simulink model "JOINTS_SPACE"  (R2021a)
settings: Solver=FixedStepAuto  StartTime=0.0  StopTime=30  FixedStep=0.01  RelTol=1e-3
model workspace: external: MATLAB File D:\OneDrive\STUDY\RIC LAB\PROJECT 6DOF\CODE\CODE 6DOF\10_SIMSCAPE\03\ROBOT_DataFile.m (data not in the file)
values from neighbouring files (symbols this model uses):
  circle = zeros(10/step+1,7)    [CIRCLE_01.m]
undefined symbols (not defined in the file or in its folder): smiData, X, Y, Z
libraries: sm_lib x36, nesl_utility x8
(part 1 of 2)
settings Model: Creator=TMP  LastModifiedBy=TMP
settings DataIOCC: SaveTime=off  ReturnWorkspaceOutputs=off

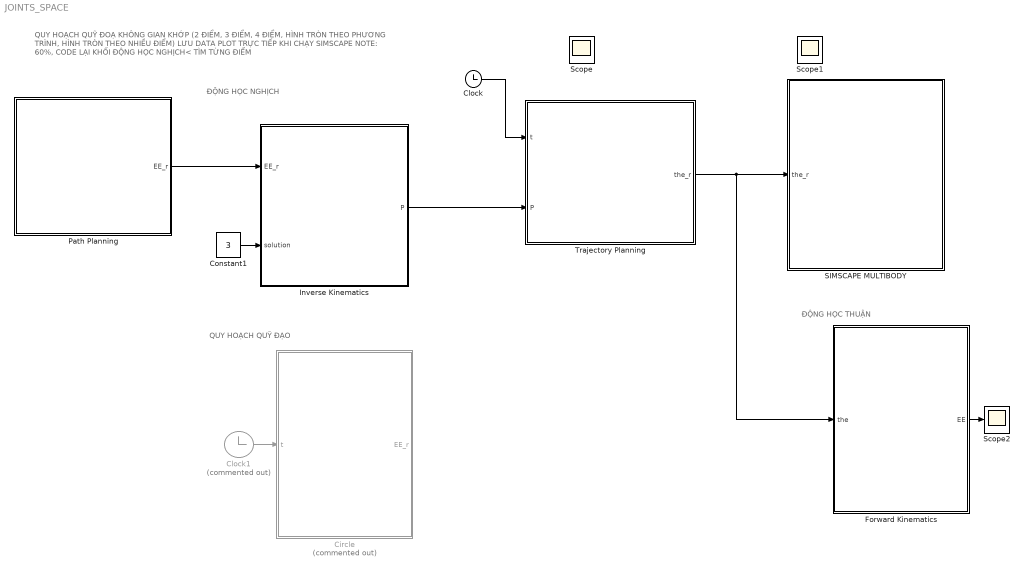
== system JOINTS_SPACE ==
  note: QUY HOẠCH QUỸ ĐOẠ KHÔNG GIAN KHỚP (2 ĐIỂM, 3 ĐIỂM, 4 ĐIỂM, HÌNH TRÒN THEO PHƯƠNG TRÌNH, HÌNH TRÒN THEO NHIỀU ĐIỂM)
      | LƯU DATA PLOT TRỰC TIẾP KHI CHẠY SIMSCAPE
      | NOTE: 60%, CODE LẠI KHỐI ĐỘNG HỌC NGHỊCH< TÌM TỪNG ĐIỂM
  note: ĐỘNG HỌC NGHỊCH
  note: QUY HOẠCH QUỸ ĐẠO
  note: ĐỘNG HỌC THUẬN
  Circle : MATLAB Function  Commented=on  TreatAsAtomicUnit=on
  Clock : Clock
  Clock1 : Clock  Commented=on
  Constant1 : Constant  Value=3
  Forward Kinematics : MATLAB Function  TreatAsAtomicUnit=on
  Inverse Kinematics : MATLAB Function  TreatAsAtomicUnit=on
  Path Planning : Subsystem
  SIMSCAPE MULTIBODY : Subsystem
  Scope : Scope
  Scope1 : Scope
  Scope2 : Scope
  Trajectory Planning : MATLAB Function  TreatAsAtomicUnit=on
  wires:
  Clock/1 -> Trajectory Planning/1(t)
  Constant1/1 -> Inverse Kinematics/2(solution)
  Clock1/1 -> Circle/1(t)
  Forward Kinematics/1(EE) -> Scope2/1
  Trajectory Planning/1(the_r) -> Forward Kinematics/1(the), SIMSCAPE MULTIBODY/1(the_r)
  Path Planning/1(EE_r) -> Inverse Kinematics/1(EE_r)
  Inverse Kinematics/1(P) -> Trajectory Planning/2(P)

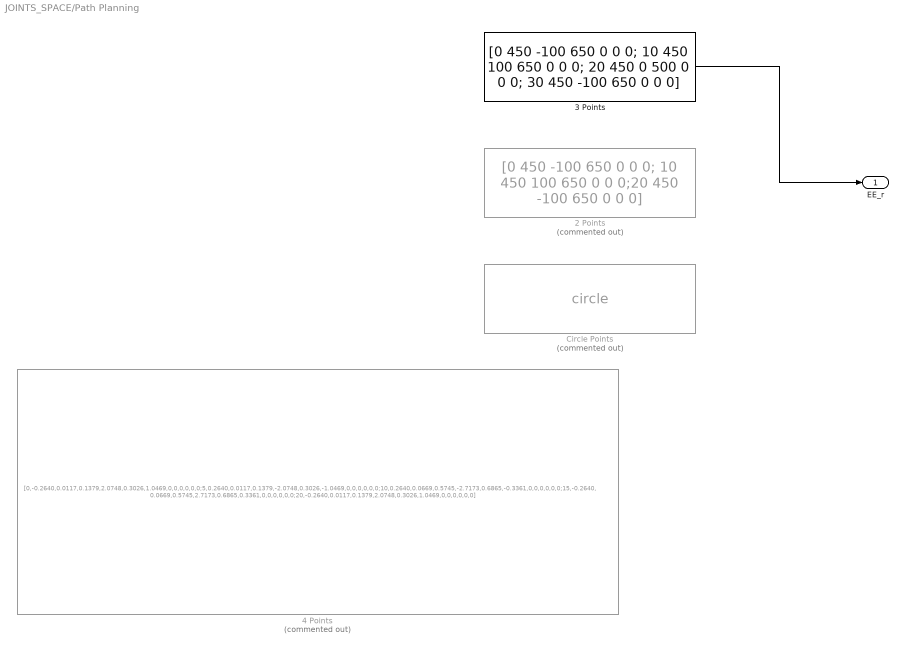
== system JOINTS_SPACE/Path Planning ==
  2 Points : Constant  Commented=on  Value=[0 450 -100 650 0 0 0; 10 450 100 650 0 0 0;20 450 -100 650 0 0 0]
  3 Points : Constant  Value=[0 450 -100 650 0 0 0; 10 450 100 650 0 0 0; 20 450 0 500 0 0 0; 30 450 -100 650 0 0 0]
  4 Points : Constant  Commented=on  Value=[0,-0.2640,0.0117,0.1379,2.0748,0.3026,1.0469,0,0,0,0,0,0;5,0.2640,0.0117,0.1379,-2.0748,0.3026,-1.0469,0,0,0,0,0,0;10,0.2640,0.0669,0.5745,-2.7173,0.6865,-0.3361,0,0,0,0,0,0;15,-0.2640, 0.0669,0.5745,2.7173,0.6865,0.3361,0,0,0,0,0,0;20,-0.2640,0.0117,0.1379,2.0748,0.3026,1.0469,0,0,0,0,0,0]
  Circle Points : Constant  Commented=on  Value=circle
  EE_r : Outport
  wires:
  3 Points/1 -> EE_r/1

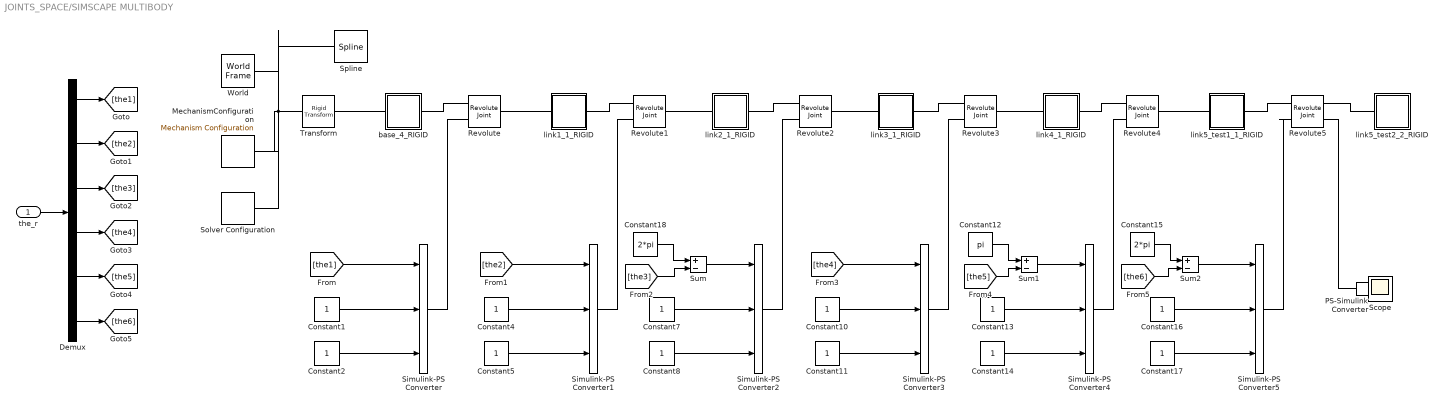
== system JOINTS_SPACE/SIMSCAPE MULTIBODY ==
  the_r : Inport
  Constant{1..2,4..5,7..8,10..11,13..14,16..17} (12 alike) : Constant
  Constant12 : Constant  Value=pi
  Constant15 : Constant  Value=2*pi
  Constant18 : Constant  Value=2*pi
  Demux : Demux  Outputs=6
  MechanismConfiguration : sm_lib/Utilities/Mechanism Configuration  UniformGravity=Constant  GravityVector=[0 -9.80665 0]  GravityVectorUnits=m/s^2  GravityUnits=m/s^2  LinearizationDelta=0.001  JointModeTransitionNonlinearIterations=2
  PS-Simulink Converter : nesl_utility/PS-Simulink Converter  PhysicalDomain=network_engine_domain  SubClassName=ps_output  LeftPortType=input  RightPortType=output  PseudoPeriodic=off  Frequencies=[]  Unit=inherit  AffineConversion=off
      settings: SourceProductBaseCode=PW,SS
  Revolute : sm_lib/Joints/Revolute Joint  JointMode=Normal  SenseConstraintForce=off  SenseConstraintForceX=off  SenseConstraintForceY=off  SenseConstraintForceZ=off  SenseConstraintTorque=off  SenseConstraintTorqueX=off  SenseConstraintTorqueY=off  SenseConstraintTorqueZ=off  SenseTotalForce=off  SenseTotalForceX=off  SenseTotalForceY=off  SenseTotalForceZ=off  SenseTotalTorque=off  SenseTotalTorqueX=off  SenseTotalTorqueY=off  SenseTotalTorqueZ=off  CompositeWrenchDir=FollowerOnBase  CompositeWrenchFrame=BaseFrame  EquilibriumPosition=0  EquilibriumPositionUnits=deg  SpringStiffness=0  SpringStiffnessUnits=N*m/deg  DampingCoefficient=0  DampingCoefficientUnits=N*m/(deg/s)  TorqueActuationMode=ComputedTorque  MotionActuationMode=InputMotion  SensePosition=off  SenseVelocity=off  SenseAcceleration=off  SenseTorqueForce=off  SenseLowerLimitTorqueForce=off  SenseUpperLimitTorqueForce=off  LowerLimitSpecify=off  LowerLimitBound=-90  LowerLimitBoundUnits=deg  LowerLimitStiffness=1e4  LowerLimitStiffnessUnits=N*m/deg  LowerLimitDamping=10  LowerLimitDampingUnits=N*m/(deg/s)  LowerLimitTransitionRegionWidth=0.1  LowerLimitTransitionRegionWidthUnits=deg  UpperLimitSpecify=off  UpperLimitBound=90  UpperLimitBoundUnits=deg  UpperLimitStiffness=1e4  UpperLimitStiffnessUnits=N*m/deg  UpperLimitDamping=10  UpperLimitDampingUnits=N*m/(deg/s)  UpperLimitTransitionRegionWidth=0.1  UpperLimitTransitionRegionWidthUnits=deg  PositionTargetSpecify=on  PositionTargetPriority=Low  PositionTargetValue=smiData.RevoluteJoint(2).Rz.Pos  PositionTargetValueUnits=deg  VelocityTargetSpecify=off  VelocityTargetPriority=High  VelocityTargetValue=0  VelocityTargetValueUnits=deg/s
  Revolute1 : sm_lib/Joints/Revolute Joint  JointMode=Normal  SenseConstraintForce=off  SenseConstraintForceX=off  SenseConstraintForceY=off  SenseConstraintForceZ=off  SenseConstraintTorque=off  SenseConstraintTorqueX=off  SenseConstraintTorqueY=off  SenseConstraintTorqueZ=off  SenseTotalForce=off  SenseTotalForceX=off  SenseTotalForceY=off  SenseTotalForceZ=off  SenseTotalTorque=off  SenseTotalTorqueX=off  SenseTotalTorqueY=off  SenseTotalTorqueZ=off  CompositeWrenchDir=FollowerOnBase  CompositeWrenchFrame=BaseFrame  EquilibriumPosition=0  EquilibriumPositionUnits=deg  SpringStiffness=0  SpringStiffnessUnits=N*m/deg  DampingCoefficient=0  DampingCoefficientUnits=N*m/(deg/s)  TorqueActuationMode=ComputedTorque  MotionActuationMode=InputMotion  SensePosition=off  SenseVelocity=off  SenseAcceleration=off  SenseTorqueForce=off  SenseLowerLimitTorqueForce=off  SenseUpperLimitTorqueForce=off  LowerLimitSpecify=off  LowerLimitBound=-90  LowerLimitBoundUnits=deg  LowerLimitStiffness=1e4  LowerLimitStiffnessUnits=N*m/deg  LowerLimitDamping=10  LowerLimitDampingUnits=N*m/(deg/s)  LowerLimitTransitionRegionWidth=0.1  LowerLimitTransitionRegionWidthUnits=deg  UpperLimitSpecify=off  UpperLimitBound=90  UpperLimitBoundUnits=deg  UpperLimitStiffness=1e4  UpperLimitStiffnessUnits=N*m/deg  UpperLimitDamping=10  UpperLimitDampingUnits=N*m/(deg/s)  UpperLimitTransitionRegionWidth=0.1  UpperLimitTransitionRegionWidthUnits=deg  PositionTargetSpecify=on  PositionTargetPriority=Low  PositionTargetValue=smiData.RevoluteJoint(1).Rz.Pos  PositionTargetValueUnits=deg  VelocityTargetSpecify=off  VelocityTargetPriority=High  VelocityTargetValue=0  VelocityTargetValueUnits=deg/s
  Revolute2 : sm_lib/Joints/Revolute Joint  JointMode=Normal  SenseConstraintForce=off  SenseConstraintForceX=off  SenseConstraintForceY=off  SenseConstraintForceZ=off  SenseConstraintTorque=off  SenseConstraintTorqueX=off  SenseConstraintTorqueY=off  SenseConstraintTorqueZ=off  SenseTotalForce=off  SenseTotalForceX=off  SenseTotalForceY=off  SenseTotalForceZ=off  SenseTotalTorque=off  SenseTotalTorqueX=off  SenseTotalTorqueY=off  SenseTotalTorqueZ=off  CompositeWrenchDir=FollowerOnBase  CompositeWrenchFrame=BaseFrame  EquilibriumPosition=0  EquilibriumPositionUnits=deg  SpringStiffness=0  SpringStiffnessUnits=N*m/deg  DampingCoefficient=0  DampingCoefficientUnits=N*m/(deg/s)  TorqueActuationMode=ComputedTorque  MotionActuationMode=InputMotion  SensePosition=off  SenseVelocity=off  SenseAcceleration=off  SenseTorqueForce=off  SenseLowerLimitTorqueForce=off  SenseUpperLimitTorqueForce=off  LowerLimitSpecify=off  LowerLimitBound=-90  LowerLimitBoundUnits=deg  LowerLimitStiffness=1e4  LowerLimitStiffnessUnits=N*m/deg  LowerLimitDamping=10  LowerLimitDampingUnits=N*m/(deg/s)  LowerLimitTransitionRegionWidth=0.1  LowerLimitTransitionRegionWidthUnits=deg  UpperLimitSpecify=off  UpperLimitBound=90  UpperLimitBoundUnits=deg  UpperLimitStiffness=1e4  UpperLimitStiffnessUnits=N*m/deg  UpperLimitDamping=10  UpperLimitDampingUnits=N*m/(deg/s)  UpperLimitTransitionRegionWidth=0.1  UpperLimitTransitionRegionWidthUnits=deg  PositionTargetSpecify=on  PositionTargetPriority=Low  PositionTargetValue=smiData.RevoluteJoint(3).Rz.Pos  PositionTargetValueUnits=deg  VelocityTargetSpecify=off  VelocityTargetPriority=High  VelocityTargetValue=0  VelocityTargetValueUnits=deg/s
  Revolute3 : sm_lib/Joints/Revolute Joint  JointMode=Normal  SenseConstraintForce=off  SenseConstraintForceX=off  SenseConstraintForceY=off  SenseConstraintForceZ=off  SenseConstraintTorque=off  SenseConstraintTorqueX=off  SenseConstraintTorqueY=off  SenseConstraintTorqueZ=off  SenseTotalForce=off  SenseTotalForceX=off  SenseTotalForceY=off  SenseTotalForceZ=off  SenseTotalTorque=off  SenseTotalTorqueX=off  SenseTotalTorqueY=off  SenseTotalTorqueZ=off  CompositeWrenchDir=FollowerOnBase  CompositeWrenchFrame=BaseFrame  EquilibriumPosition=0  EquilibriumPositionUnits=deg  SpringStiffness=0  SpringStiffnessUnits=N*m/deg  DampingCoefficient=0  DampingCoefficientUnits=N*m/(deg/s)  TorqueActuationMode=ComputedTorque  MotionActuationMode=InputMotion  SensePosition=off  SenseVelocity=off  SenseAcceleration=off  SenseTorqueForce=off  SenseLowerLimitTorqueForce=off  SenseUpperLimitTorqueForce=off  LowerLimitSpecify=off  LowerLimitBound=-90  LowerLimitBoundUnits=deg  LowerLimitStiffness=1e4  LowerLimitStiffnessUnits=N*m/deg  LowerLimitDamping=10  LowerLimitDampingUnits=N*m/(deg/s)  LowerLimitTransitionRegionWidth=0.1  LowerLimitTransitionRegionWidthUnits=deg  UpperLimitSpecify=off  UpperLimitBound=90  UpperLimitBoundUnits=deg  UpperLimitStiffness=1e4  UpperLimitStiffnessUnits=N*m/deg  UpperLimitDamping=10  UpperLimitDampingUnits=N*m/(deg/s)  UpperLimitTransitionRegionWidth=0.1  UpperLimitTransitionRegionWidthUnits=deg  PositionTargetSpecify=on  PositionTargetPriority=Low  PositionTargetValue=smiData.RevoluteJoint(4).Rz.Pos  PositionTargetValueUnits=deg  VelocityTargetSpecify=off  VelocityTargetPriority=High  VelocityTargetValue=0  VelocityTargetValueUnits=deg/s
  Revolute4 : sm_lib/Joints/Revolute Joint  JointMode=Normal  SenseConstraintForce=off  SenseConstraintForceX=off  SenseConstraintForceY=off  SenseConstraintForceZ=off  SenseConstraintTorque=off  SenseConstraintTorqueX=off  SenseConstraintTorqueY=off  SenseConstraintTorqueZ=off  SenseTotalForce=off  SenseTotalForceX=off  SenseTotalForceY=off  SenseTotalForceZ=off  SenseTotalTorque=off  SenseTotalTorqueX=off  SenseTotalTorqueY=off  SenseTotalTorqueZ=off  CompositeWrenchDir=FollowerOnBase  CompositeWrenchFrame=BaseFrame  EquilibriumPosition=0  EquilibriumPositionUnits=deg  SpringStiffness=0  SpringStiffnessUnits=N*m/deg  DampingCoefficient=0  DampingCoefficientUnits=N*m/(deg/s)  TorqueActuationMode=ComputedTorque  MotionActuationMode=InputMotion  SensePosition=off  SenseVelocity=off  SenseAcceleration=off  SenseTorqueForce=off  SenseLowerLimitTorqueForce=off  SenseUpperLimitTorqueForce=off  LowerLimitSpecify=off  LowerLimitBound=-90  LowerLimitBoundUnits=deg  LowerLimitStiffness=1e4  LowerLimitStiffnessUnits=N*m/deg  LowerLimitDamping=10  LowerLimitDampingUnits=N*m/(deg/s)  LowerLimitTransitionRegionWidth=0.1  LowerLimitTransitionRegionWidthUnits=deg  UpperLimitSpecify=off  UpperLimitBound=90  UpperLimitBoundUnits=deg  UpperLimitStiffness=1e4  UpperLimitStiffnessUnits=N*m/deg  UpperLimitDamping=10  UpperLimitDampingUnits=N*m/(deg/s)  UpperLimitTransitionRegionWidth=0.1  UpperLimitTransitionRegionWidthUnits=deg  PositionTargetSpecify=on  PositionTargetPriority=Low  PositionTargetValue=smiData.RevoluteJoint(5).Rz.Pos  PositionTargetValueUnits=deg  VelocityTargetSpecify=off  VelocityTargetPriority=High  VelocityTargetValue=0  VelocityTargetValueUnits=deg/s
  Revolute5 : sm_lib/Joints/Revolute Joint  JointMode=Normal  SenseConstraintForce=off  SenseConstraintForceX=off  SenseConstraintForceY=off  SenseConstraintForceZ=off  SenseConstraintTorque=off  SenseConstraintTorqueX=off  SenseConstraintTorqueY=off  SenseConstraintTorqueZ=off  SenseTotalForce=off  SenseTotalForceX=off  SenseTotalForceY=off  SenseTotalForceZ=off  SenseTotalTorque=off  SenseTotalTorqueX=off  SenseTotalTorqueY=off  SenseTotalTorqueZ=off  CompositeWrenchDir=FollowerOnBase  CompositeWrenchFrame=BaseFrame  EquilibriumPosition=0  EquilibriumPositionUnits=deg  SpringStiffness=0  SpringStiffnessUnits=N*m/deg  DampingCoefficient=0  DampingCoefficientUnits=N*m/(deg/s)  TorqueActuationMode=ComputedTorque  MotionActuationMode=InputMotion  SensePosition=on  SenseVelocity=off  SenseAcceleration=off  SenseTorqueForce=off  SenseLowerLimitTorqueForce=off  SenseUpperLimitTorqueForce=off  LowerLimitSpecify=off  LowerLimitBound=-90  LowerLimitBoundUnits=deg  LowerLimitStiffness=1e4  LowerLimitStiffnessUnits=N*m/deg  LowerLimitDamping=10  LowerLimitDampingUnits=N*m/(deg/s)  LowerLimitTransitionRegionWidth=0.1  LowerLimitTransitionRegionWidthUnits=deg  UpperLimitSpecify=off  UpperLimitBound=90  UpperLimitBoundUnits=deg  UpperLimitStiffness=1e4  UpperLimitStiffnessUnits=N*m/deg  UpperLimitDamping=10  UpperLimitDampingUnits=N*m/(deg/s)  UpperLimitTransitionRegionWidth=0.1  UpperLimitTransitionRegionWidthUnits=deg  PositionTargetSpecify=on  PositionTargetPriority=Low  PositionTargetValue=smiData.RevoluteJoint(6).Rz.Pos  PositionTargetValueUnits=deg  VelocityTargetSpecify=off  VelocityTargetPriority=High  VelocityTargetValue=0  VelocityTargetValueUnits=deg/s
  Scope : Scope
  Simulink-PS Converter{,1..5} (6 alike) : nesl_utility/Simulink-PS Converter  PhysicalDomain=network_engine_domain  SubClassName=ps_input  LeftPortType=input  RightPortType=output  PseudoPeriodic=off  Frequencies=[]  NoiseDistribution=none  NoiseParameters=[]  Unit=1  AffineConversion=off  FilteringAndDerivatives=provide  SimscapeFilterOrder=1  InputFilterTimeConstant=0.001  UdotUserProvided=2
      settings: SourceProductBaseCode=PW,SS
  Solver Configuration : nesl_utility/Solver Configuration  PhysicalDomain=network_engine_domain  SubClassName=solver  LeftPortType=input  RightPortType=generic  Tones=[]  Harmonics=[]  SimulateNoise=off  Profile=off  UseLocalSampling=off  EnableSwitchedLinearOptims=on  FrequencyDomain=off  UseCCode=off  RelTol=0.001  AbsTol=1e-06  MinStep=1e-09  ToWorkspace=off  RevertToSquareIcSolve=off  NumHomotopyIterations=100  PhasorMode=off  PhasorModeNumHarmonics=1  DoDC=off  ResidualTolerance=1e-09  UseLocalSolver=off  LocalSolverChoice=NE_BACKWARD_EULER_ADVANCER  LocalSolverSampleTime=0.001  DoFixedCost=off  MaxNonlinIter=3  MaxModeIter=2  ComputeImpulses=off  ImpulseIterations=2  LinearAlgebra=auto  EquationFormulation=NE_TIME_EF  DelaysMemoryBudget=1024  AutomaticFiltering=on  FilteringTimeConstant=0.001  PartitionStorageMethod=AS_NEEDED  PartitionMemoryBudget=1024  PartitionMethod=ROBUST
      settings: SourceProductBaseCode=PW,SS
  Spline : sm_lib/Curves and Surfaces/Spline  GraphicAmbientColor=[0.15 0.15 0.15 1.0]  GraphicDiffuseColor=[0.0 0.0 0.0]  DataPoints=|  DataPointsUnits=mm  GraphicEmissiveColor=[0.0 0.0 0.0 1.0]  EndConditionType=Natural  MarkerShape=Sphere  MarkerSize=10  GraphicType=FromGeometry  GraphicOpacity=1.0  GraphicShininess=75  GraphicSpecularColor=[0.5 0.5 0.5 1.0]  GraphicVisPropType=SimpleVisualProperties
      | [450.0000 -100.0000  650.0000
      |   450.0025  -99.9863  649.9959
      |   450.0101  -99.9452  649.9836
      |   450.0226  -99.8770  649.9633
      |   450.0400  -99.7820  649.9349
      |   450.0623  -99.6603  649.8985
      |   450.0893  -99.5124  649.8541
      |   450.1211  -99.3383  649.8018
      |   450.1574  -99.1384  649.7416
      |   450.1982  -98.9130  649.6736
      |   450.2434  -98.6623  649.5977
      |   450.2929  -98.3867  649.5141
      |   450.3465  -98.0864  649.4226
      |   450.4043  -97.7618  649.3234
      |   450.4659  -97.4131  649.2165
      |   450.5313  -97.0408  649.1017
      |   450.6004  -96.6450  648.9793
      |   450.6730  -96.2262  648.8491
      |   450.7490  -95.7847  648.7113
      |   450.8283  -95.3209  648.5657
      |   450.9106  -94.8350  648.4124
      |   450.9958  -94.3276  648.2514
      |   451.0837  -93.7988  648.0827
      |   451.1743  -93.2491  647.9063
      |   451.2673  -92.6789  647.7223
      |   451.3626  -92.0886  647.5305
      |   451.4600  -91.4785  647.3311
      |   451.5593  -90.8490  647.1240
      |   451.6604  -90.2006  646.9093
      |   451.7631  -89.5337  646.6869
      |   451.8672  -88.8486  646.4570
      |   451.9725  -88.1458  646.2194
      |   452.0789  -87.4257  645.9743
      |   452.1862  -86.6887  645.7216
      |   452.2942  -85.9353  645.4614
      |   452.4027  -85.1659  645.1937
      |   452.5117  -84.3810  644.9186
      |   452.6208  -83.5809  644.6361
      |   452.7300  -82.7662  644.3462
      |   452.8390  -81.9372  644.0491
      |   452.9478  -81.0945  643.7447
      |   453.0561  -80.2385  643.4332
      |   453.1637  -79.3697  643.1146
      |   453.2706  -78.4885  642.7891
      |   453.3766  -77.5954  642.4566
      |   453.4815  -76.6908  642.1173
      |   453.5851  -75.7753  641.7713
      |   453.6874  -74.8494  641.4188
      |   453.7882  -73.9134  641.0598
      |   453.8874  -72.9678  640.6944
      |   453.9847  -72.0133  640.3228
      |   454.0802  -71.0501  639.9452
      |   454.1737  -70.0788  639.5617
      |   454.2650  -69.0999  639.1725
      |   454.3542  -68.1138  638.7777
      |   454.4410  -67.1210  638.3775
      |   454.5253  -66.1219  637.9721
      |   454.6072  -65.1171  637.5618
      |   454.6864  -64.1070  637.1466
      |   454.7630  -63.0921  636.7270
      |   454.8368  -62.0728  636.3029
      |   454.9078  -61.0495  635.8748
      |   454.9759  -60.0228  635.4428
      |   455.0412  -58.9930  635.0073
      |   455.1034  -57.9605  634.5684
      |   455.1627  -56.9259  634.1264
      |   455.2190  -55.8895  633.6817
      |   455.2722  -54.8517  633.2345
      |   455.3223  -53.8130  632.7851
      |   455.3694  -52.7737  632.3338
      |   455.4134  -51.7343  631.8810
      |   455.4544  -50.6950  631.4269
      |   455.4923  -49.6563  630.9719
      |   455.5272  -48.6185  630.5163
      |   455.5591  -47.5820  630.0605
      |   455.5881  -46.5471  629.6048
      |   455.6141  -45.5141  629.1496
      |   455.6373  -44.4833  628.6952
      |   455.6576  -43.4551  628.2420
      |   455.6752  -42.4296  627.7904
      |   455.6901  -41.4073  627.3407
      |   455.7023  -40.3883  626.8933
      |   455.7121  -39.3728  626.4487
      |   455.7193  -38.3611  626.0072
      |   455.7242  -37.3535  625.5691
      |   455.7268  -36.3501  625.1349
      |   455.7273  -35.3510  624.7050
      |   455.7256  -34.3565  624.2798
      |   455.7220  -33.3667  623.8596
      |   455.7164  -32.3818  623.4448
      |   455.7092  -31.4018  623.0359
      |   455.7003  -30.4269  622.6333
      |   455.6898  -29.4571  622.2372
      |   455.6779  -28.4925  621.8481
      |   455.6648  -27.5332  621.4665
      |   455.6504  -26.5792  621.0926
      |   455.6350  -25.6305  620.7268
      |   455.6187  -24.6872  620.3696
      |   455.6016  -23.7491  620.0212
      |   455.5838  -22.8164  619.6820
      |   455.5655  -21.8888  619.3525
      |   455.5467  -20.9665  619.0328
      |   455.5276  -20.0493  618.7234
      |   455.5084  -19.1371  618.4246
      |   455.4890  -18.2298  618.1367
      |   455.4697  -17.3273  617.8600
      |   455.4505  -16.4295  617.5948
      |   455.4316  -15.5363  617.3414
      |   455.4131  -14.6473  617.1001
      |   455.3950  -13.7626  616.8711
      |   455.3775  -12.8819  616.6546
      |   455.3607  -12.0050  616.4510
      |   455.3446  -11.1318  616.2604
      |   455.3294  -10.2619  616.0831
      |   455.3150   -9.3952  615.9192
      |   455.3017   -8.5315  615.7689
      |   455.2894   -7.6705  615.6325
      |   455.2783   -6.8119  615.5100
      |   455.2683   -5.9555  615.4015
      |   455.2595   -5.1011  615.3073
      |   455.2521   -4.2483  615.2274
      |   455.2459   -3.3970  615.1619
      |   455.2411   -2.5467  615.1109
      |   455.2376   -1.6974  615.0744
      |   455.2355   -0.8485  615.0525
      |   455.2348   -0.0000  615.0452
      |   455.2355    0.8485  615.0525
      |   455.2376    1.6974  615.0744
      |   455.2411    2.5467  615.1109
      |   455.2459    3.3970  615.1619
      |   455.2521    4.2483  615.2274
      |   455.2595    5.1011  615.3073
      |   455.2683    5.9555  615.4015
      |   455.2783    6.8119  615.5100
      |   455.2894    7.6705  615.6325
      |   455.3017    8.5315  615.7689
      |   455.3150    9.3952  615.9192
      |   455.3294   10.2619  616.0831
      |   455.3446   11.1318  616.2604
      |   455.3607   12.0050  616.4510
      |   455.3775   12.8819  616.6546
      |   455.3950   13.7626  616.8711
      |   455.4131   14.6473  617.1001
      |   455.4316   15.5363  617.3414
      |   455.4505   16.4295  617.5948
      |   455.4697   17.3273  617.8600
      |   455.4890   18.2298  618.1367
      |   455.5084   19.1371  618.4246
      |   455.5276   20.0493  618.7234
      |   455.5467   20.9665  619.0328
      |   455.5655   21.8888  619.3525
      |   455.5838   22.8164  619.6820
      |   455.6016   23.7491  620.0212
      |   455.6187   24.6872  620.3696
      |   455.6350   25.6305  620.7268
      |   455.6504   26.5792  621.0926
      |   455.6648   27.5332  621.4665
      |   455.6779   28.4925  621.8481
      |   455.6898   29.4571  622.2372
      |   455.7003   30.4269  622.6333
      |   455.7092   31.4018  623.0359
      |   455.7164   32.3818  623.4448
      |   455.7220   33.3667  623.8596
      |   455.7256   34.3565  624.2798
      |   455.7273   35.3510  624.7050
      |   455.7268   36.3501  625.1349
      |   455.7242   37.3535  625.5691
      |   455.7193   38.3611  626.0072
      |   455.7121   39.3728  626.4487
      |   455.7023   40.3883  626.8933
      |   455.6901   41.4073  627.3407
      |   455.6752   42.4296  627.7904
      |   455.6576   43.4551  628.2420
      |   455.6373   44.4833  628.6952
      |   455.6141   45.5141  629.1496
      |   455.5881   46.5471  629.6048
      |   455.5591   47.5820  630.0605
      |   455.5272   48.6185  630.5163
      |   455.4923   49.6563  630.9719
      |   455.4544   50.6950  631.4269
      |   455.4134   51.7343  631.8810
      |   455.3694   52.7737  632.3338
      |   455.3223   53.8130  632.7851
      |   455.2722   54.8517  633.2345
      |   455.2190   55.8895  633.6817
      |   455.1627   56.9259  634.1264
      |   455.1034   57.9605  634.5684
      |   455.0412   58.9930  635.0073
      |   454.9759   60.0228  635.4428
      |   454.9078   61.0495  635.8748
      |   454.8368   62.0728  636.3029
      |   454.7630   63.0921  636.7270
      |   454.6864   64.1070  637.1466
      |   454.6072   65.1171  637.5618
      |   454.5253   66.1219  637.9721
      |   454.4410   67.1210  638.3775
      |   454.3542   68.1138  638.7777
      |   454.2650   69.0999  639.1725
      |   454.1737   70.0788  639.5617
      |   454.0802   71.0501  639.9452
      |   453.9847   72.0133  640.3228
      |   453.8874   72.9678  640.6944
      |   453.7882   73.9134  641.0598
      |   453.6874   74.8494  641.4188
      |   453.5851   75.7753  641.7713
      |   453.4815   76.6908  642.1173
      |   453.3766   77.5954  642.4566
      |   453.2706   78.4885  642.7891
      |   453.1637   79.3697  643.1146
      |   453.0561   80.2385  643.4332
      |   452.9478   81.0945  643.7447
      |   452.8390   81.9372  644.0491
      |   452.7300   82.7662  644.3462
      |   452.6208   83.5809  644.6361
      |   452.5117   84.3810  644.9186
      |   452.4027   85.1659  645.1937
      |   452.2942   85.9353  645.4614
      |   452.1862   86.6887  645.7216
      |   452.0789   87.4257  645.9743
      |   451.9725   88.1458  646.2194
      |   451.8672   88.8486  646.4570
      |   451.7631   89.5337  646.6869
      |   451.6604   90.2006  646.9093
      |   451.5593   90.8490  647.1240
      |   451.4600   91.4785  647.3311
      |   451.3626   92.0886  647.5305
      |   451.2673   92.6789  647.7223
      |   451.1743   93.2491  647.9063
      |   451.0837   93.7988  648.0827
      |   450.9958   94.3276  648.2514
      |   450.9106   94.8350  648.4124
      |   450.8283   95.3209  648.5657
      |   450.7490   95.7847  648.7113
      |   450.6730   96.2262  648.8491
      |   450.6004   96.6450  648.9793
      |   450.5313   97.0408  649.1017
      |   450.4659   97.4131  649.2165
      |   450.4043   97.7618  649.3234
      |   450.3465   98.0864  649.4226
      |   450.2929   98.3867  649.5141
      |   450.2434   98.6623  649.5977
      |   450.1982   98.9130  649.6736
      |   450.1574   99.1384  649.7416
      |   450.1211   99.3383  649.8018
      |   450.0893   99.5124  649.8541
      |   450.0623   99.6603  649.8985
      |   450.0400   99.7820  649.9349
      |   450.0226   99.8770  649.9633
      |   450.0101   99.9452  649.9836
      |   450.0025   99.9863  649.9959
      |   450.0000  100.0000  650.0000
      |   450.0024   99.9905  649.9865
      |   450.0095   99.9621  649.9460
      |   450.0212   99.9150  649.8788
      |   450.0376   99.8494  649.7850
      |   450.0584   99.7654  649.6648
      |   450.0837   99.6633  649.5183
      |   450.1133   99.5431  649.3458
      |   450.1471   99.4053  649.1473
      |   450.1850   99.2499  648.9230
      |   450.2268   99.0771  648.6729
      |   450.2725   98.8873  648.3972
      |   450.3217   98.6807  648.0959
      |   450.3745   98.4575  647.7691
      |   450.4306   98.2179  647.4170
      |   450.4898   97.9623  647.0395
      |   450.5519   97.6910  646.6367
      |   450.6167   97.4041  646.2087
      |   450.6841   97.1021  645.7555
      |   450.7538   96.7852  645.2771
      |   450.8255   96.4538  644.7736
      |   450.8991   96.1081  644.2451
      |   450.9743   95.7486  643.6915
      |   451.0509   95.3755  643.1128
      |   451.1285   94.9893  642.5091
      |   451.2069   94.5903  641.8805
      |   451.2860   94.1789  641.2269
      |   451.3652   93.7555  640.5483
      |   451.4445   93.3205  639.8449
      |   451.5235   92.8743  639.1166
      |   451.6018   92.4174  638.3634
      |   451.6793   91.9503  637.5854
      |   451.7556   91.4733  636.7827
      |   451.8303   90.9869  635.9553
      |   451.9032   90.4917  635.1032
      |   451.9740   89.9881  634.2266
      |   452.0423   89.4767  633.3255
      |   452.1077   88.9579  632.4000
      |   452.1701   88.4323  631.4501
      |   452.2290   87.9005  630.4761
      |   452.2841   87.3631  629.4780
      |   452.3351   86.8205  628.4560
      |   452.3816   86.2734  627.4102
      |   452.4234   85.7224  626.3408
      |   452.4600   85.1680  625.2480
      |   452.4913   84.6110  624.1320
      |   452.5167   84.0520  622.9930
      |   452.5361   83.4915  621.8313
      |   452.5490   82.9303  620.6471
      |   452.5553   82.3689  619.4407
      |   452.5545   81.8082  618.2124
      |   452.5464   81.2486  616.9626
      |   452.5307   80.6910  615.6916
      |   452.5071   80.1361  614.3998
      |   452.4753   79.5844  613.0876
      |   452.4351   79.0368  611.7554
      |   452.3862   78.4939  610.4037
      |   452.3283   77.9564  609.0330
      |   452.2613   77.4250  607.6438
      |   452.1848   76.9005  606.2365
      |   452.0988   76.3835  604.8119
      |   452.0030   75.8748  603.3704
      |   451.8972   75.3750  601.9127
      |   451.7813   74.8849  600.4394
      |   451.6551   74.4051  598.9513
      |   451.5186   73.9363  597.4490
      |   451.3715   73.4792  595.9332
      |   451.2140   73.0345  594.4048
      |   451.0458   72.6027  592.8645
      |   450.8669   72.1846  591.3131
      |   450.6774   71.7808  589.7515
      |   450.4772   71.3918  588.1805
      |   450.2663   71.0183  586.6011
      |   450.0449   70.6607  585.0141
      |   449.8130   70.3197  583.4205
      |   449.5707   69.9958  581.8213
      |   449.3181   69.6895  580.2175
      |   449.0554   69.4011  578.6100
      |   448.7827   69.1313  576.9999
      |   448.5003   68.8803  575.3883
      |   448.2085   68.6486  573.7761
      |   447.9074   68.4365  572.1645
      |   447.5974   68.2443  570.5546
      |   447.2787   68.0722  568.9475
      |   446.9518   67.9206  567.3443
      |   446.6170   67.7897  565.7461
      |   446.2746   67.6794  564.1541
      |   445.9251   67.5901  562.5693
      |   445.5690   67.5218  560.9930
      |   445.2067   67.4744  559.4263
      |   444.8386   67.4480  557.8702
      |   444.4654   67.4426  556.3260
      |   444.0876   67.4579  554.7947
      |   443.7056   67.4939  553.2776
      |   443.3201   67.5504  551.7756
      |   442.9318   67.6271  550.2899
      |   442.5411   67.7237  548.8216
      |   442.1488   67.8399  547.3718
      |   441.7554   67.9752  545.9414
      |   441.3617   68.1293  544.5315
      |   440.9683   68.3016  543.1432
      |   440.5759   68.4916  541.7773
      |   440.1852   68.6988  540.4349
      |   439.7969   68.9224  539.1169
      |   439.4117   69.1618  537.8240
      |   439.0303   69.4163  536.5572
      |   438.6534   69.6851  535.3174
      |   438.2818   69.9674  534.1051
      |   437.9162   70.2623  532.9213
      |   437.5572   70.5689  531.7665
      |   437.2055   70.8864  530.6415
      |   436.8620   71.2136  529.5467
      |   436.5272   71.5497  528.4829
      |   436.2018   71.8935  527.4503
      |   435.8865   72.2440  526.4496
      |   435.5819   72.6001  525.4811
      |   435.2888   72.9607  524.5452
      |   435.0076   73.3245  523.6421
      |   434.7389   73.6904  522.7720
      |   434.4834   74.0571  521.9353
      |   434.2416   74.4236  521.1319
      |   434.0140   74.7885  520.3620
      |   433.8011   75.1505  519.6256
      |   433.6034   75.5085  518.9226
      |   433.4212   75.8611  518.2530
      |   433.2550   76.2070  517.6166
      |   433.1052   76.5451  517.0132
      |   432.9720   76.8741  516.4425
      |   432.8558   77.1925  515.9043
      |   432.7569   77.4994  515.3980
      |   432.6754   77.7932  514.9235
      |   432.6115   78.0730  514.4801
      |   432.5655   78.3373  514.0673
      |   432.5373   78.5851  513.6846
      |   432.5271   78.8151  513.3314
      |   432.5348   79.0263  513.0070
      |   432.5605   79.2175  512.7107
      |   432.6041   79.3876  512.4417
      |   432.6655   79.5355  512.1993
      |   432.7446   79.6603  511.9827
      |   432.8411   79.7610  511.7909
      |   432.9550   79.8367  511.6232
      |   433.0859   79.8864  511.4786
      |   433.2334   79.9093  511.3561
      |   433.3974   79.9047  511.2547
      |   433.5775   79.8717  511.1736
      |   433.7731   79.8098  511.1116
      |   433.9840   79.7181  511.0677
      |   434.2096   79.5963  511.0409
      |   434.4494   79.4437  511.0301
      |   434.7029   79.2598  511.0343
      |   434.9696   79.0443  511.0523
      |   435.2488   78.7968  511.0831
      |   435.5400   78.5169  511.1255
      |   435.8425   78.2046  511.1786
      |   436.1557   77.8595  511.2412
      |   436.4788   77.4817  511.3123
      |   436.8113   77.0709  511.3908
      |   437.1524   76.6273  511.4756
      |   437.5014   76.1509  511.5656
      |   437.8575   75.6418  511.6600
      |   438.2201   75.1003  511.7576
      |   438.5884   74.5265  511.8575
      |   438.9615   73.9208  511.9586
      |   439.3389   73.2836  512.0602
      |   439.7197   72.6152  512.1611
      |   440.1031   71.9162  512.2607
      |   440.4885   71.1870  512.3579
      |   440.8751   70.4283  512.4520
      |   441.2621   69.6406  512.5422
      |   441.6488   68.8247  512.6277
      |   442.0345   67.9813  512.7079
      |   442.4186   67.1111  512.7819
      |   442.8002   66.2149  512.8492
      |   443.1788   65.2937  512.9092
      |   443.5537   64.3483  512.9612
      |   443.9243   63.3796  513.0048
      |   444.2899   62.3885  513.0395
      |   444.6499   61.3762  513.0648
      |   445.0039   60.3435  513.0803
      |   445.3512   59.2916  513.0856
      |   445.6914   58.2215  513.0805
      |   446.0239   57.1343  513.0646
      |   446.3483   56.0311  513.0377
      |   446.6642   54.9131  512.9995
      |   446.9711   53.7814  512.9501
      |   447.2688   52.6372  512.8891
      |   447.5567   51.4816  512.8166
      |   447.8348   50.3158  512.7324
      |   448.1026   49.1411  512.6367
      |   448.3599   47.9585  512.5294
      |   448.6065   46.7693  512.4107
      |   448.8423   45.5748  512.2805
      |   449.0671   44.3759  512.1392
      |   449.2807   43.1741  511.9868
      |   449.4830   41.9703  511.8235
      |   449.6742   40.7659  511.6497
      |   449.8540   39.5620  511.4656
      |   450.0225   38.3597  511.2715
      |   450.1797   37.1601  511.0677
      |   450.3257   35.9644  510.8547
      |   450.4607   34.7738  510.6327
      |   450.5846   33.5892  510.4022
      |   450.6977   32.4118  510.1636
      |   450.8001   31.2426  509.9175
      |   450.8921   30.0827  509.6642
      |   450.9738   28.9330  509.4043
      |   451.0456   27.7946  509.1383
      |   451.1075   26.6685  508.8667
      |   451.1601   25.5556  508.5900
      |   451.2035   24.4568  508.3088
      |   451.2380   23.3731  508.0237
      |   451.2641   22.3052  507.7353
      |   451.2821   21.2542  507.4441
      |   451.2923   20.2207  507.1508
      |   451.2952   19.2057  506.8558
      |   451.2911   18.2098  506.5600
      |   451.2805   17.2339  506.2638
      |   451.2637   16.2787  505.9678
      |   451.2412   15.3449  505.6727
      |   451.2134   14.4333  505.3791
      |   451.1808   13.5443  505.0877
      |   451.1438   12.6788  504.7989
      |   451.1029   11.8374  504.5134
      |   451.0584   11.0206  504.2319
      |   451.0109   10.2290  503.9548
      |   450.9608    9.4631  503.6829
      |   450.9085    8.7237  503.4166
      |   450.8545    8.0110  503.1566
      |   450.7993    7.3257  502.9034
      |   450.7431    6.6683  502.6575
      |   450.6865    6.0392  502.4196
      |   450.6299    5.4389  502.1900
      |   450.5737    4.8677  501.9694
      |   450.5183    4.3262  501.7583
      |   450.4640    3.8148  501.5570
      |   450.4113    3.3338  501.3661
      |   450.3604    2.8837  501.1861
      |   450.3118    2.4648  501.0173
      |   450.2657    2.0775  500.8602
      |   450.2225    1.7222  500.7152
      |   450.1824    1.3992  500.5826
      |   450.1457    1.1088  500.4628
      |   450.1127    0.8514  500.3561
      |   450.0835    0.6273  500.2629
      |   450.0585    0.4369  500.1833
      |   450.0377    0.2804  500.1178
      |   450.0213    0.1582  500.0665
      |   450.0095    0.0705  500.0297
      |   450.0024    0.0177  500.0074
      |   450.0000    0.0000  500.0000
      |   450.0024   -0.0032  500.0074
      |   450.0095   -0.0129  500.0297
      |   450.0214   -0.0290  500.0666
      |   450.0380   -0.0514  500.1181
      |   450.0591   -0.0801  500.1840
      |   450.0848   -0.1150  500.2643
      |   450.1151   -0.1562  500.3588
      |   450.1498   -0.2035  500.4673
      |   450.1889   -0.2570  500.5898
      |   450.2324   -0.3166  500.7261
      |   450.2801   -0.3822  500.8761
      |   450.3320   -0.4539  501.0397
      |   450.3881   -0.5315  501.2168
      |   450.4482   -0.6151  501.4072
      |   450.5124   -0.7047  501.6108
      |   450.5805   -0.8002  501.8274
      |   450.6524   -0.9015  502.0571
      |   450.7281   -1.0087  502.2996
      |   450.8075   -1.1217  502.5547
      |   450.8905   -1.2406  502.8225
      |   450.9771   -1.3652  503.1027
      |   451.0671   -1.4956  503.3952
      |   451.1604   -1.6317  503.7000
      |   451.2571   -1.7735  504.0168
      |   451.3569   -1.9211  504.3455
      |   451.4598   -2.0743  504.6861
      |   451.5657   -2.2333  505.0383
      |   451.6746   -2.3978  505.4021
      |   451.7863   -2.5680  505.7773
      |   451.9007   -2.7439  506.1638
      |   452.0177   -2.9253  506.5615
      |   452.1373   -3.1123  506.9702
      |   452.2594   -3.3049  507.3898
      |   452.3838   -3.5031  507.8202
      |   452.5104   -3.7069  508.2612
      |   452.6393   -3.9162  508.7128
      |   452.7701   -4.1310  509.1748
      |   452.9030   -4.3513  509.6470
      |   453.0377   -4.5772  510.1293
      |   453.1742   -4.8086  510.6216
      |   453.3124   -5.0454  511.1238
      |   453.4521   -5.2878  511.6357
      |   453.5933   -5.5356  512.1572
      |   453.7359   -5.7889  512.6882
      |   453.8798   -6.0476  513.2286
      |   454.0249   -6.3118  513.7781
      |   454.1710   -6.5814  514.3367
      |   454.3181   -6.8564  514.9043
      |   454.4662   -7.1368  515.4807
      |   454.6150   -7.4227  516.0657
      |   454.7645   -7.7139  516.6593
      |   454.9146   -8.0105  517.2614
      |   455.0651   -8.3125  517.8717
      |   455.2161   -8.6199  518.4902
      |   455.3675   -8.9326  519.1167
      |   455.5190   -9.2506  519.7512
      |   455.6706   -9.5739  520.3934
      |   455.8223   -9.9026  521.0432
      |   455.9739  -10.2366  521.7006
      |   456.1254  -10.5759  522.3653
      |   456.2766  -10.9204  523.0373
      |   456.4274  -11.2702  523.7164
      |   456.5779  -11.6252  524.4025
      |   456.7278  -11.9855  525.0954
      |   456.8771  -12.3510  525.7951
      |   457.0257  -12.7216  526.5015
      |   457.1736  -13.0975  527.2142
      |   457.3206  -13.4785  527.9334
      |   457.4667  -13.8647  528.6588
      |   457.6117  -14.2560  529.3902
      |   457.7556  -14.6523  530.1277
      |   457.8984  -15.0538  530.8710
      |   458.0398  -15.4603  531.6200
      |   458.1800  -15.8719  532.3746
      |   458.3187  -16.2885  533.1347
      |   458.4559  -16.7100  533.9001
      |   458.5915  -17.1365  534.6708
      |   458.7255  -17.5680  535.4465
      |   458.8578  -18.0044  536.2272
      |   458.9883  -18.4456  537.0128
      |   459.1170  -18.8917  537.8031
      |   459.2437  -19.3427  538.5981
      |   459.3685  -19.7984  539.3975
      |   459.4912  -20.2588  540.2013
      |   459.6118  -20.7240  541.0093
      |   459.7302  -21.1939  541.8215
      |   459.8464  -21.6684  542.6377
      |   459.9602  -22.1476  543.4577
      |   460.0718  -22.6313  544.2816
      |   460.1809  -23.1196  545.1091
      |   460.2875  -23.6123  545.9401
      |   460.3917  -24.1095  546.7746
      |   460.4932  -24.6111  547.6124
      |   460.5922  -25.1171  548.4534
      |   460.6884  -25.6274  549.2974
      |   460.7820  -26.1420  550.1444
      |   460.8728  -26.6608  550.9943
      |   460.9608  -27.1837  551.8469
      |   461.0459  -27.7108  552.7022
      |   461.1282  -28.2420  553.5599
      |   461.2075  -28.7772  554.4201
      |   461.2839  -29.3163  555.2826
      |   461.3572  -29.8594  556.1472
      |   461.4276  -30.4062  557.0140
      |   461.4948  -30.9569  557.8826
      |   461.5589  -31.5113  558.7532
      |   461.6199  -32.0694  559.6255
      |   461.6778  -32.6311  560.4995
      |   461.7324  -33.1963  561.3750
      |   461.7839  -33.7649  562.2519
      |   461.8321  -34.3370  563.1301
      |   461.8770  -34.9124  564.0096
      |   461.9187  -35.4911  564.8902
      |   461.9570  -36.0730  565.7718
      |   461.9920  -36.6580  566.6543
      |   462.0237  -37.2460  567.5376
      |   462.0521  -37.8370  568.4216
      |   462.0770  -38.4308  569.3062
      |   462.0986  -39.0275  570.1914
      |   462.1169  -39.6270  571.0769
      |   462.1317  -40.2290  571.9627
      |   462.1431  -40.8337  572.8487
      |   462.1511  -41.4408  573.7347
      |   462.1557  -42.0503  574.6208
      |   462.1569  -42.6621  575.5068
      |   462.1547  -43.2761  576.3925
      |   462.1491  -43.8923  577.2780
      |   462.1401  -44.5105  578.1630
      |   462.1277  -45.1307  579.0475
      |   462.1118  -45.7527  579.9314
      |   462.0926  -46.3764  580.8146
      |   462.0700  -47.0018  581.6970
      |   462.0441  -47.6288  582.5785
      |   462.0147  -48.2573  583.4590
      |   461.9821  -48.8871  584.3384
      |   461.9461  -49.5182  585.2165
      |   461.9068  -50.1504  586.0934
      |   461.8642  -50.7837  586.9689
      |   461.8183  -51.4180  587.8429
      |   461.7692  -52.0531  588.7152
      |   461.7169  -52.6889  589.5859
      |   461.6614  -53.3254  590.4548
      |   461.6026  -53.9624  591.3217
      |   461.5408  -54.5999  592.1867
      |   461.4758  -55.2376  593.0496
      |   461.4077  -55.8755  593.9103
      |   461.3366  -56.5135  594.7687
      |   461.2625  -57.1515  595.6247
      |   461.1853  -57.7893  596.4782
      |   461.1053  -58.4269  597.3291
      |   461.0223  -59.0641  598.1773
      |   460.9364  -59.7008  599.0227
      |   460.8478  -60.3369  599.8652
      |   460.7563  -60.9723  600.7047
      |   460.6621  -61.6068  601.5411
      |   460.5652  -62.2403  602.3742
      |   460.4657  -62.8728  603.2041
      |   460.3635  -63.5040  604.0306
      |   460.2589  -64.1339  604.8535
      |   460.1517  -64.7624  605.6728
      |   460.0421  -65.3893  606.4884
      |   459.9301  -66.0145  607.3001
      |   459.8158  -66.6378  608.1079
      |   459.6992  -67.2593  608.9117
      |   459.5805  -67.8786  609.7113
      |   459.4595  -68.4958  610.5066
      |   459.3365  -69.1106  611.2976
      |   459.2115  -69.7230  612.0841
      |   459.0845  -70.3328  612.8660
      |   458.9556  -70.9400  613.6432
      |   458.8249  -71.5443  614.4156
      |   458.6924  -72.1457  615.1831
      |   458.5583  -72.7440  615.9455
      |   458.4225  -73.3391  616.7029
      |   458.2852  -73.9309  617.4549
      |   458.1465  -74.5192  618.2016
      |   458.0063  -75.1039  618.9429
      |   457.8648  -75.6850  619.6785
      |   457.7221  -76.2622  620.4084
      |   457.5783  -76.8355  621.1325
      |   457.4333  -77.4046  621.8507
      |   457.2874  -77.9696  622.5628
      |   457.1406  -78.5303  623.2687
      |   456.9929  -79.0865  623.9684
      |   456.8445  -79.6381  624.6616
      |   456.6954  -80.1850  625.3483
      |   456.5457  -80.7270  626.0284
      |   456.3956  -81.2641  626.7017
      |   456.2450  -81.7961  627.3681
      |   456.0942  -82.3230  628.0275
      |   455.9431  -82.8444  628.6798
      |   455.7919  -83.3605  629.3248
      |   455.6406  -83.8709  629.9625
      |   455.4894  -84.3757  630.5927
      |   455.3384  -84.8746  631.2152
      |   455.1875  -85.3676  631.8300
      |   455.0371  -85.8546  632.4370
      |   454.8870  -86.3353  633.0359
      |   454.7374  -86.8098  633.6268
      |   454.5885  -87.2778  634.2094
      |   454.4403  -87.7393  634.7836
      |   454.2929  -88.1941  635.3493
      |   454.1464  -88.6422  635.9064
      |   454.0009  -89.0833  636.4548
      |   453.8564  -89.5175  636.9943
      |   453.7132  -89.9445  637.5248
      |   453.5713  -90.3642  638.0462
      |   453.4308  -90.7766  638.5583
      |   453.2917  -91.1815  639.0610
      |   453.1542  -91.5789  639.5542
      |   453.0184  -91.9685  640.0377
      |   452.8844  -92.3503  640.5115
      |   452.7523  -92.7242  640.9754
      |   452.6221  -93.0900  641.4293
      |   452.4940  -93.4477  641.8730
      |   452.3681  -93.7971  642.3064
      |   452.2444  -94.1381  642.7294
      |   452.1230  -94.4707  643.1418
      |   452.0042  -94.7946  643.5435
      |   451.8878  -95.1099  643.9345
      |   451.7741  -95.4163  644.3145
      |   451.6631  -95.7138  644.6834
      |   451.5550  -96.0023  645.0412
      |   451.4497  -96.2816  645.3876
      |   451.3474  -96.5518  645.7226
      |   451.2483  -96.8125  646.0459
      |   451.1523  -97.0638  646.3576
      |   451.0595  -97.3056  646.6574
      |   450.9702  -97.5377  646.9453
      |   450.8842  -97.7600  647.2210
      |   450.8017  -97.9725  647.4845
      |   450.7229  -98.1749  647.7357
      |   450.6477  -98.3674  647.9743
      |   450.5763  -98.5496  648.2004
      |   450.5087  -98.7216  648.4137
      |   450.4450  -98.8831  648.6142
      |   450.3853  -99.0342  648.8016
      |   450.3296  -99.1748  648.9760
      |   450.2780  -99.3046  649.1371
      |   450.2306  -99.4237  649.2848
      |   450.1875  -99.5319  649.4191
      |   450.1487  -99.6291  649.5397
      |   450.1142  -99.7152  649.6466
      |   450.0842  -99.7902  649.7397
      |   450.0587  -99.8539  649.8187
      |   450.0377  -99.9063  649.8837
      |   450.0213  -99.9471  649.9344
      |   450.0095  -99.9764  649.9708
      |   450.0024  -99.9941  649.9927
      |   450.0000 -100.0000  650.0000]
  Sum : Sum  Inputs=+-
  Sum1 : Sum  Inputs=+-
  Sum2 : Sum  Inputs=+-
  Transform : sm_lib/Frames and Transforms/Rigid Transform  TranslationMethod=Cartesian  TranslationStandardOffset=0  TranslationLengthUnit=mm  TranslationStandardAxis=+Z  TranslationCartesianOffset=smiData.RigidTransform(13).translation  TranslationROffset=0  TranslationROffsetUnits=m  TranslationZOffset=0  TranslationZOffsetUnits=m  TranslationThetaOffset=0  TranslationThetaOffsetUnits=deg  RotationMethod=ArbitraryAxis  RotationAngleUnits=rad  RotationStandardAxis=+Z  RotationAngle=smiData.RigidTransform(13).angle  RotationArbitraryAxis=smiData.RigidTransform(13).axis  FollAlignAxisA=+X  BaseAlignAxisA=+Y  FollAlignAxisB=+Y  BaseAlignAxisB=+Z  RotationSequenceAxes=FollowerAxes  RotationSequence=XYX  RotationSequenceAngles=[0 0 0]  RotationSequenceAnglesUnits=deg  RotationMatrix=[1 0 0; 0 1 0; 0 0 1]
  World : sm_lib/Frames and Transforms/World Frame
  base_4_RIGID : Subsystem
  link1_1_RIGID : Subsystem
  link2_1_RIGID : Subsystem
  link3_1_RIGID : Subsystem
  link4_1_RIGID : Subsystem
  link5_test1_1_RIGID : Subsystem
  link5_test2_2_RIGID : Subsystem
  wires:
  [the2] -> Simulink-PS Converter1/1
  Sum2/1 -> Simulink-PS Converter5/1
  [the4] -> Simulink-PS Converter3/1
  Constant17/1 -> Simulink-PS Converter5/3
  Constant12/1 -> Sum1/1
  Constant5/1 -> Simulink-PS Converter1/3
  Constant7/1 -> Simulink-PS Converter2/2
  [the6] -> Sum2/2
  Constant1/1 -> Simulink-PS Converter/2
  Sum1/1 -> Simulink-PS Converter4/1
  Constant13/1 -> Simulink-PS Converter4/2
  Sum/1 -> Simulink-PS Converter2/1
  Constant15/1 -> Sum2/1
  Constant16/1 -> Simulink-PS Converter5/2
  Constant11/1 -> Simulink-PS Converter3/3
  Constant10/1 -> Simulink-PS Converter3/2
  [the5] -> Sum1/2
  [the3] -> Sum/2
  Constant18/1 -> Sum/1
  [the1] -> Simulink-PS Converter/1
  Constant2/1 -> Simulink-PS Converter/3
  Constant4/1 -> Simulink-PS Converter1/2
  Constant14/1 -> Simulink-PS Converter4/3
  Constant8/1 -> Simulink-PS Converter2/3
  the_r/1 -> Demux/1
  Demux/1 -> [the1]
  Demux/2 -> [the2]
  Demux/3 -> [the3]
  Demux/4 -> [the4]
  Demux/5 -> [the5]
  Demux/6 -> [the6]
  PS-Simulink Converter/1 -> Scope/1
  connections:
  Revolute5/LConn1 -- link5_test1_1_RIGID/RConn1
  Revolute2/LConn1 -- link2_1_RIGID/RConn1
  MechanismConfiguration/RConn1 -- Solver Configuration/RConn1 -- World/RConn1 -- Spline/LConn1 -- Transform/LConn1
  Simulink-PS Converter/RConn1 -- Revolute/LConn2
  Revolute5/RConn1 -- link5_test2_2_RIGID/LConn1
  Revolute/RConn1 -- link1_1_RIGID/LConn1
  Revolute1/LConn1 -- link1_1_RIGID/RConn1
  Revolute3/LConn2 -- Simulink-PS Converter3/RConn1
  Revolute2/RConn1 -- link3_1_RIGID/LConn1
  Revolute1/RConn1 -- link2_1_RIGID/LConn1
  Revolute4/RConn1 -- link5_test1_1_RIGID/LConn1
  Revolute3/LConn1 -- link3_1_RIGID/RConn1
  Revolute4/LConn1 -- link4_1_RIGID/RConn1
  Revolute/LConn1 -- base_4_RIGID/RConn1
  Revolute4/LConn2 -- Simulink-PS Converter4/RConn1
  Revolute3/RConn1 -- link4_1_RIGID/LConn1
  Revolute2/LConn2 -- Simulink-PS Converter2/RConn1
  Revolute1/LConn2 -- Simulink-PS Converter1/RConn1
  Revolute5/LConn2 -- Simulink-PS Converter5/RConn1
  PS-Simulink Converter/LConn1 -- Revolute5/RConn2
  Transform/RConn1 -- base_4_RIGID/LConn1

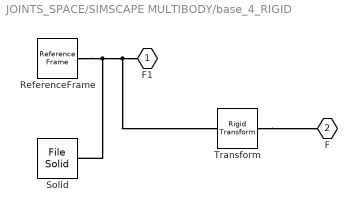
== system JOINTS_SPACE/SIMSCAPE MULTIBODY/base_4_RIGID ==
  ReferenceFrame : sm_lib/Frames and Transforms/Reference Frame
  Solid : sm_lib/Body Elements/File Solid  ExtGeomFileName=base_Default_sldprt.STEP  UnitType=FromFile  ExtGeomFileUnits=m  StepReaderType=HEX  ExportConvexHullGeometry=off  InertiaType=Custom  Mass=smiData.Solid(5).mass  MassUnits=kg  CenterOfMass=smiData.Solid(5).CoM  CenterOfMassUnits=mm  MomentsOfInertia=smiData.Solid(5).MoI  MomentsOfInertiaUnits=kg*mm^2  ProductsOfInertia=smiData.Solid(5).PoI  ProductsOfInertiaUnits=kg*mm^2  BasedOnType=DensityFromFile  Density=1000  DensityUnits=kg/m^3  DoExposeReferenceFrame=on  SerializedFrames=<Frames/>  GraphicType=FromGeometry  MarkerShape=Sphere  MarkerSize=10  GraphicVisPropType=SimpleVisualProperties  GraphicDiffuseColor=smiData.Solid(5).color  GraphicSpecularColor=[0.5 0.5 0.5 1.0]  GraphicAmbientColor=[0.15 0.15 0.15 1.0]  GraphicEmissiveColor=[0.0 0.0 0.0 1.0]  GraphicShininess=75  GraphicOpacity=smiData.Solid(5).opacity
  Transform : sm_lib/Frames and Transforms/Rigid Transform  TranslationMethod=Cartesian  TranslationStandardOffset=0  TranslationLengthUnit=mm  TranslationStandardAxis=+Z  TranslationCartesianOffset=smiData.RigidTransform(3).translation  TranslationROffset=0  TranslationROffsetUnits=m  TranslationZOffset=0  TranslationZOffsetUnits=m  TranslationThetaOffset=0  TranslationThetaOffsetUnits=deg  RotationMethod=ArbitraryAxis  RotationAngleUnits=rad  RotationStandardAxis=+Z  RotationAngle=smiData.RigidTransform(3).angle  RotationArbitraryAxis=smiData.RigidTransform(3).axis  FollAlignAxisA=+X  BaseAlignAxisA=+Y  FollAlignAxisB=+Y  BaseAlignAxisB=+Z  RotationSequenceAxes=FollowerAxes  RotationSequence=XYX  RotationSequenceAngles=[0 0 0]  RotationSequenceAnglesUnits=deg  RotationMatrix=[1 0 0; 0 1 0; 0 0 1]
  F1 : PMIOPort  Side=Left
  F : PMIOPort  Port=2  Side=Right
  connections:
  Solid/RConn1 -- ReferenceFrame/RConn1 -- Transform/LConn1 -- F1/RConn1
  Transform/RConn1 -- F/RConn1
